simulink model "Group15_Final_Demo_Code"  (R2023a)
settings: Solver=FixedStepAuto  StartTime=0.0  StopTime=inf  FixedStep=0.00001  RelTol=1e-3
undefined symbols (not defined in the file): DiscIntNeverNeededParam
libraries: arduinolib x14, simulink x3, hdlsllib x2, mobileRoboticsTrainingLib x1, arduinosensorlib x1
settings Model: NumberOfSteps=50  PacingRate=1000  ExtModeTrigDuration=2  Creator=Boitumelo  LastModifiedBy=jana
settings OptimizationCC: EnhancedBackFolding=on  PassReuseOutputArgsAs=Individual arguments  ZeroExternalMemoryAtStartup=off  ZeroInternalMemoryAtStartup=off  MaxStackSize=64  OptimizeBlockOrder=speed  DifferentSizesBufferReuse=on  OptimizationCustomize=off  EfficientTunableParamExpr=on
settings DebuggingCC: ParameterTunabilityLossMsg=error  UnconnectedInputMsg=warning  UnconnectedOutputMsg=warning  UnconnectedLineMsg=warning  UnderSpecifiedDimensionMsg=warning
settings HardwareCC: ProdBitPerPointer=32  ProdBitPerSizeT=32  ProdBitPerPtrDiffT=32  ProdLargestAtomicInteger=Long  ProdLargestAtomicFloat=Double  ProdWordSize=32  ProdHWDeviceType=ARM Compatible->ARM Cortex  UseEmbeddedCoderFeatures=off  UseSimulinkCoderFeatures=off
settings ModelReferenceCC: EnableRefExpFcnMdlSchedulingChecks=on
settings SFSimCC: MATLABDynamicMemAlloc=off
settings RTWCC: Description=Embedded Coder  SystemTargetFile=ert.tlc  HardwareBoard=Arduino Nano 33 IoT  TemplateMakefile=ert_default_tmf  Toolchain=Arduino ARM  BuildConfiguration=Faster Runs  DLArmComputeVersion=19.05
settings CodeAppCC: ForceParamTrailComments=on  IgnoreCustomStorageClasses=off  OperatorAnnotations=on  SimulinkDataObjDesc=on  SFDataObjDesc=on  InsertBlockDesc=on
settings ERTTargetCC: SupportContinuousTime=on  SupportNonInlinedSFcns=on  SupportVariableSizeSignals=on  ExtModeTransport=2  ExtModeStaticAlloc=on  ExtModeAutomaticAllocSize=off  ExtModeStaticAllocSize=8192  ExtModeMexFile=ext_xcp  ExtModeIntrfLevel=Level2 - Open

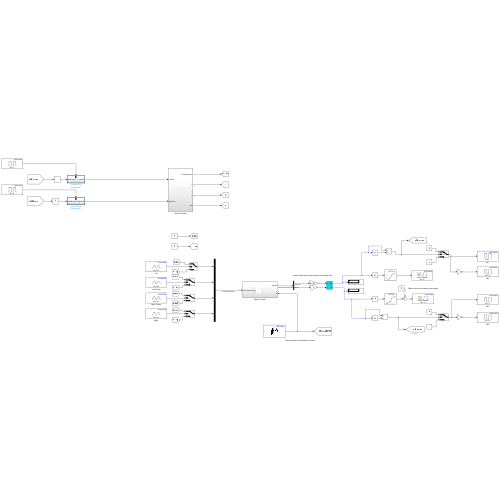
[thumbnail: Simulink's stored preview of the top-level diagram]
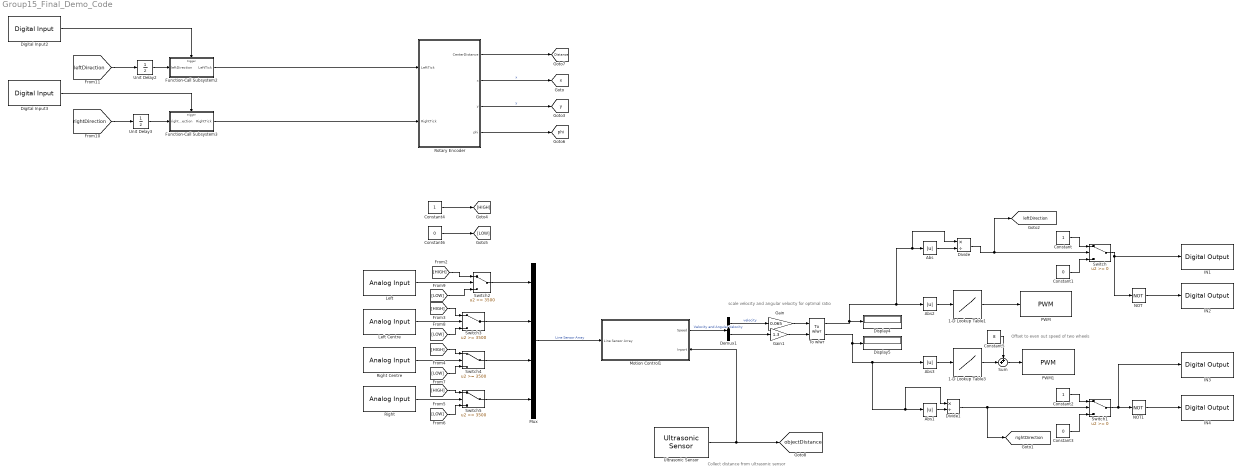
== system Group15_Final_Demo_Code ==
  note: Offset to even out speed of two wheels
  note: Collect distance from ultrasonic sensor
  note: scale velocity and angular velocity for optimal ratio
  1-D Lookup Table1 : Lookup_n-D  NumberOfTableDimensions=1  BreakpointsForDimension1=[-12.5105278523077 -12.3751973907692 -12.2398669292308 -12.1045364676923 -11.9692060061538 -11.8338755446154 -11.6985450830769 -11.5632146215385 -11.42788416 -11.2925536984615 -11.1572232369231 -11.0218927753846 -10.8865623138461 -10.7512318523077 -10.6159013907692 -10.4805709292308 -10.3452404676923 -10.2099100061538 -10.0745795446154 -9.93924908307692 -9.80391862153846 -9.66858816 -9.53325769846154 -9.39792723692308 -9.26259677538462 -9.12726631384615 -8.99193585230769 -8.85660539076923 -8.72127492923077 -8.58594446769231 -8.45061400615385 -8.31528354461539 -8.17995308307692 -8.04462262153846 -7.90929216 -7.77396169846154 -7.63863123692308 -7.50330077538462 -7.36797031384615 -7.23263985230769 -7.09730939076923 -6.96197892923077 -6.82664846769231 -6.69131800615385 -6.55598754461539 -6.42065708307692 -6.28532662153846 -6.14999616 -6.01466569846154 -5.87933523692308 -5.74400477538462 -5.60867431384616 -5.47334385230769 -5.33801339076923 -5.20268292923077 -5.06735246769231 -4.93202200615385 -4.79669154461538 -4.66136108307692 -4.52603062153846 -4.39070016 -4.303992 -4.178328 -4.021248 -3.832752 -3.644256 -3.518592 -3.45576 -3.330096 -3.204432 -3.015936 -2.890272 -2.764608 -2.576112 -2.51328 -2.3562 -2.167704 -2.136288 -1.916376 -1.790712 -1.633632 -1.5708 -1.445136 -1.350888 -1.162392 -1.005312 0 1.005312 1.162392 1.350888 1.445136 1.5708 1.633632 1.790712 1.916376 2.136288 2.167704 2.3562 2.51328 2.576112 2.764608 2.890272 3.015936 3.204432 3.330096 3.45576 3.518592 3.644256 3.832752 4.021248 4.178328 4.303992 4.39070016 4.52603062153846 4.66136108307692 4.79669154461538 4.93202200615384 5.06735246769231 5.20268292923077 5.33801339076923 5.47334385230769 5.60867431384615 5.74400477538461 5.87933523692307 6.01466569846154 6.14999616 6.28532662153846 6.42065708307692 6.55598754461538 6.69131800615384 6.8266484676923 6.96197892923077 7.09730939076923 7.23263985230769 7.36797031384615 7.50330077538461 7.63863123692307 7.77396169846154 7.90929216 8.04462262153846 8.17995308307692 8.31528354461538 8.45061400615384 8.5859444676923 8.72127492923077 8.85660539076923 8.99193585230769 9.12726631384615 9.26259677538461 9.39792723692307 9.53325769846153 9.66858816 9.80391862153846 9.93924908307692 10.0745795446154 10.2099100061538 10.3452404676923 10.4805709292308 10.6159013907692 10.7512318523077 10.8865623138462 11.0218927753847 11.1572232369231 11.2925536984616 11.42788416 11.5632146215385 11.698545083077 11.8338755446154 11.9692060061539 12.1045364676923 12.2398669292308 12.3751973907693 12.5105278523077]  Table=[-127 -126 -125 -124 -123 -122 -121 -120 -119 -118 -117 -116 -115 -114 -113 -112 -111 -110 -109 -108 -107 -106 -105 -104 -103 -102 -101 -100 -99 -98 -97 -96 -95 -94 -93 -92 -91 -90 -89 -88 -87 -86 -85 -84 -83 -82 -81 -80 -79 -78 -77 -76 -75 -74 -73 -72 -71 -70 -69 -68 -67 -66 -65 -64 -63 -62 -61 -60 -59 -58 -57 -56 -55 -54 -53 -52 -51 -50 -49 -48 -47 -46 -45 -44 -43 -42 0 42 43 44 45 46 47 48 49 50 51 52 53 54 55 56 57 58 59 60 61 62 63 64 65 66 67 68 69 70 71 72 73 74 75 76 77 78 79 80 81 82 83 84 85 86 87 88 89 90 91 92 93 94 95 96 97 98 99 100 101 102 103 104 105 106 107 108 109 110 111 112 113 114 115 116 117 118 119 120 121 122 123 124 125 126 127]  InternalRulePriority=Speed  RndMeth=Simplest
  1-D Lookup Table3 : Lookup_n-D  NumberOfTableDimensions=1  BreakpointsForDimension1=[-12.5105278523077 -12.3751973907692 -12.2398669292308 -12.1045364676923 -11.9692060061538 -11.8338755446154 -11.6985450830769 -11.5632146215385 -11.42788416 -11.2925536984615 -11.1572232369231 -11.0218927753846 -10.8865623138461 -10.7512318523077 -10.6159013907692 -10.4805709292308 -10.3452404676923 -10.2099100061538 -10.0745795446154 -9.93924908307692 -9.80391862153846 -9.66858816 -9.53325769846154 -9.39792723692308 -9.26259677538462 -9.12726631384615 -8.99193585230769 -8.85660539076923 -8.72127492923077 -8.58594446769231 -8.45061400615385 -8.31528354461539 -8.17995308307692 -8.04462262153846 -7.90929216 -7.77396169846154 -7.63863123692308 -7.50330077538462 -7.36797031384615 -7.23263985230769 -7.09730939076923 -6.96197892923077 -6.82664846769231 -6.69131800615385 -6.55598754461539 -6.42065708307692 -6.28532662153846 -6.14999616 -6.01466569846154 -5.87933523692308 -5.74400477538462 -5.60867431384616 -5.47334385230769 -5.33801339076923 -5.20268292923077 -5.06735246769231 -4.93202200615385 -4.79669154461538 -4.66136108307692 -4.52603062153846 -4.39070016 -4.303992 -4.178328 -4.021248 -3.832752 -3.644256 -3.518592 -3.45576 -3.330096 -3.204432 -3.015936 -2.890272 -2.764608 -2.576112 -2.51328 -2.3562 -2.167704 -2.136288 -1.916376 -1.790712 -1.633632 -1.5708 -1.445136 -1.350888 -1.162392 -1.005312 0 1.005312 1.162392 1.350888 1.445136 1.5708 1.633632 1.790712 1.916376 2.136288 2.167704 2.3562 2.51328 2.576112 2.764608 2.890272 3.015936 3.204432 3.330096 3.45576 3.518592 3.644256 3.832752 4.021248 4.178328 4.303992 4.39070016 4.52603062153846 4.66136108307692 4.79669154461538 4.93202200615384 5.06735246769231 5.20268292923077 5.33801339076923 5.47334385230769 5.60867431384615 5.74400477538461 5.87933523692307 6.01466569846154 6.14999616 6.28532662153846 6.42065708307692 6.55598754461538 6.69131800615384 6.8266484676923 6.96197892923077 7.09730939076923 7.23263985230769 7.36797031384615 7.50330077538461 7.63863123692307 7.77396169846154 7.90929216 8.04462262153846 8.17995308307692 8.31528354461538 8.45061400615384 8.5859444676923 8.72127492923077 8.85660539076923 8.99193585230769 9.12726631384615 9.26259677538461 9.39792723692307 9.53325769846153 9.66858816 9.80391862153846 9.93924908307692 10.0745795446154 10.2099100061538 10.3452404676923 10.4805709292308 10.6159013907692 10.7512318523077 10.8865623138462 11.0218927753847 11.1572232369231 11.2925536984616 11.42788416 11.5632146215385 11.698545083077 11.8338755446154 11.9692060061539 12.1045364676923 12.2398669292308 12.3751973907693 12.5105278523077]  Table=[-127 -126 -125 -124 -123 -122 -121 -120 -119 -118 -117 -116 -115 -114 -113 -112 -111 -110 -109 -108 -107 -106 -105 -104 -103 -102 -101 -100 -99 -98 -97 -96 -95 -94 -93 -92 -91 -90 -89 -88 -87 -86 -85 -84 -83 -82 -81 -80 -79 -78 -77 -76 -75 -74 -73 -72 -71 -70 -69 -68 -67 -66 -65 -64 -63 -62 -61 -60 -59 -58 -57 -56 -55 -54 -53 -52 -51 -50 -49 -48 -47 -46 -45 -44 -43 -42 0 42 43 44 45 46 47 48 49 50 51 52 53 54 55 56 57 58 59 60 61 62 63 64 65 66 67 68 69 70 71 72 73 74 75 76 77 78 79 80 81 82 83 84 85 86 87 88 89 90 91 92 93 94 95 96 97 98 99 100 101 102 103 104 105 106 107 108 109 110 111 112 113 114 115 116 117 118 119 120 121 122 123 124 125 126 127]  InternalRulePriority=Speed  RndMeth=Simplest
  Abs{,1..3} (4 alike) : Abs  SaturateOnIntegerOverflow=off
  Constant : Constant
  Constant1 : Constant  Value=0
  Constant2 : Constant
  Constant3 : Constant  Value=0
  Constant4 : Constant
  Constant5 : Constant  Value=8
  Constant6 : Constant  Value=0
  Demux1 : Demux  Outputs=2
  Digital Input2 : arduinolib/Digital Input  pinNumber=3  mode=Default  Direction=input  SampleTime=0.001  blockPlatform=arduino
  Digital Input3 : arduinolib/Digital Input  pinNumber=2  mode=Default  Direction=input  SampleTime=0.001  blockPlatform=arduino
  Display4 : Display
  Display5 : Display
  Divide : Product  Inputs=*/
  Divide1 : Product  Inputs=*/
  Function-Call Subsystem2 : Subsystem  TreatAsAtomicUnit=on
  Function-Call Subsystem3 : Subsystem  TreatAsAtomicUnit=on
  Gain : Gain  Gain=0.065
  Gain1 : Gain  Gain=1.3
  IN1 : arduinolib/Digital Output  pinNumber=7  Direction=output  blockPlatform=arduino
  IN2 : arduinolib/Digital Output  pinNumber=8  Direction=output  blockPlatform=arduino
  IN3 : arduinolib/Digital Output  pinNumber=9  Direction=output  blockPlatform=arduino
  IN4 : arduinolib/Digital Output  pinNumber=10  Direction=output  blockPlatform=arduino
  Left : arduinolib/Analog Input  pinNumber=7  ReadResultsOnly=off  ConversionTriggerSource=Software  ExternalTriggerType=uint32( 0 )  OutputDataType=uint16  EnableConversionCompleteNotify=off  EnableOuputStatus=off  SampleTime=0.0001  blockPlatform=arduino
  Left Centre : arduinolib/Analog Input  pinNumber=0  ReadResultsOnly=off  ConversionTriggerSource=Software  ExternalTriggerType=uint32( 0 )  OutputDataType=uint16  EnableConversionCompleteNotify=off  EnableOuputStatus=off  SampleTime=0.0001  blockPlatform=arduino
  Motion Control1 : Subsystem
      settings: PortSchema="{\"entries\":[{\"content\":{\"sides\":[{\"content\":{\"connectorIds\":[\"In1\"]},\"type\":\"ConnectorPlacement.EquallySpacedRectSide\",\"uuid\":\"8c902054-c90d-4041-a30b-e9972f3a80fd\"},{\"content\":{\"connectorIds\":[\"Out1\",\"In2\"],\"side\":\"RIGHT\"},\"type\":\"ConnectorPlacement.EquallySpacedRectSide\",\"uuid\":\"d90cf934-ce11-4f50-afe0-98fc417ab745\"},{\"content\":{\"side\":\"TOP\"},\"type\":\"ConnectorPlacement.EquallySpacedRectSide\",\"uuid\":\"2acc5f33-e61f-44f0-84c4-b841351b747b\"}]},\"type\":\"ConnectorPlacement.EquallySpacedConnector\",\"uuid\":\"ebe61945-3866-4bce-ba54-5c93c237d4bb\"}],\"packageUris\":[\"http://schema.mathworks.com/mf0/Connector/R2020b\"],\"version\":\"1.0\"}"
  Mux : Mux
  NOT : Logic  Operator=NOT  IconShape=distinctive  AllPortsSameDT=off  OutDataTypeStr=boolean
  NOT1 : Logic  Operator=NOT  IconShape=distinctive  AllPortsSameDT=off  OutDataTypeStr=boolean
  PWM : arduinolib/PWM  pinNumber=6  frequencyType=Default  desiredFrequency=490.2  achievableFrequency=490.2
  PWM1 : arduinolib/PWM  pinNumber=11  frequencyType=Default  desiredFrequency=490.2  achievableFrequency=490.2
  Right : arduinolib/Analog Input  pinNumber=2  ReadResultsOnly=off  ConversionTriggerSource=Software  ExternalTriggerType=uint32( 0 )  OutputDataType=uint16  EnableConversionCompleteNotify=off  EnableOuputStatus=off  SampleTime=0.0001  blockPlatform=arduino
  Right Centre : arduinolib/Analog Input  pinNumber=1  ReadResultsOnly=off  ConversionTriggerSource=Software  ExternalTriggerType=uint32( 0 )  OutputDataType=uint16  EnableConversionCompleteNotify=off  EnableOuputStatus=off  SampleTime=0.0001  blockPlatform=arduino
  Rotary Encoder : Subsystem
  Sum : Sum  Inputs=++|
  Switch : Switch  SaturateOnIntegerOverflow=off  InputSameDT=off
  Switch1 : Switch  SaturateOnIntegerOverflow=off  InputSameDT=off
  Switch{2..5} (4 alike) : Switch  Threshold=3500  SaturateOnIntegerOverflow=off  InputSameDT=off
  To wlwr : mobileRoboticsTrainingLib/To wlwr  axleLength=0.17  wheelR=0.031
  Ultrasonic Sensor : arduinosensorlib/Ultrasonic Sensor  NumSignalPins=2  TrigPin=4  EchoPin=5  SignalPin=3  SampleTime_=0.05  blockPlatform=ARDUINO
  Unit Delay2 : UnitDelay  SampleTime=-1  HasFrameUpgradeWarning=on
  Unit Delay3 : UnitDelay  SampleTime=-1  HasFrameUpgradeWarning=on
  tag scope: Distance=global, leftDirection=global, objectDistance=global, phi=global, rightDirection=global, x=global, y=global
  wires:
  Mux/1 -> Motion Control1/1(Line Sensor Array)  "Line Sensor Array"
  Abs/1 -> Divide/2
  Divide/1 -> [leftDirection], Switch/2
  Divide1/1 -> [rightDirection], Switch1/2
  Abs1/1 -> Divide1/2
  Constant/1 -> Switch/1
  Switch/1 -> NOT/1, IN1/1
  Constant1/1 -> Switch/3
  NOT/1 -> IN2/1
  Constant2/1 -> Switch1/1
  Switch1/1 -> NOT1/1, IN3/1
  Constant3/1 -> Switch1/3
  NOT1/1 -> IN4/1
  [HIGH] -> Switch2/1
  [HIGH] -> Switch3/1
  [HIGH] -> Switch4/1
  [HIGH] -> Switch5/1
  [LOW] -> Switch5/3
  [LOW] -> Switch4/3
  [LOW] -> Switch3/3
  [LOW] -> Switch2/3
  Left/1 -> Switch2/2
  Right Centre/1 -> Switch4/2
  Right/1 -> Switch5/2
  Switch2/1 -> Mux/1
  Switch3/1 -> Mux/2
  Switch4/1 -> Mux/3
  Switch5/1 -> Mux/4
  Constant4/1 -> [HIGH]
  Constant6/1 -> [LOW]
  1-D Lookup Table1/1 -> PWM/1
  1-D Lookup Table3/1 -> Sum/2
  Ultrasonic Sensor/1 -> Motion Control1/2(Inport), [objectDistance]
  [rightDirection] -> Unit Delay3/1
  Unit Delay3/1 -> Function-Call Subsystem3/1(rightDirection)
  Unit Delay2/1 -> Function-Call Subsystem2/1(leftDirection)
  Rotary Encoder/3(y) -> [y]  "y"
  Rotary Encoder/2(x) -> [x]  "x"
  Digital Input3/1 -> Function-Call Subsystem3/Trigger
  Digital Input2/1 -> Function-Call Subsystem2/Trigger
  [leftDirection] -> Unit Delay2/1
  Function-Call Subsystem2/1(LeftTick) -> Rotary Encoder/1(LeftTick)
  Rotary Encoder/4(phi) -> [phi]
  Function-Call Subsystem3/1(RightTick) -> Rotary Encoder/2(RightTick)
  Left Centre/1 -> Switch3/2
  Rotary Encoder/1(CenterDistance) -> [Distance]
  To wlwr/1 -> Divide/1, Abs/1, Abs2/1, Display4/1
  To wlwr/2 -> Abs3/1, Divide1/1, Abs1/1, Display5/1
  Abs2/1 -> 1-D Lookup Table1/1
  Abs3/1 -> 1-D Lookup Table3/1
  Constant5/1 -> Sum/1
  Sum/1 -> PWM1/1
  Gain/1 -> To wlwr/1
  Gain1/1 -> To wlwr/2
  Motion Control1/1(Speed) -> Demux1/1  "Velocity and Angular Velocity"
  Demux1/2 -> Gain1/1
  Demux1/1 -> Gain/1  "velocity"

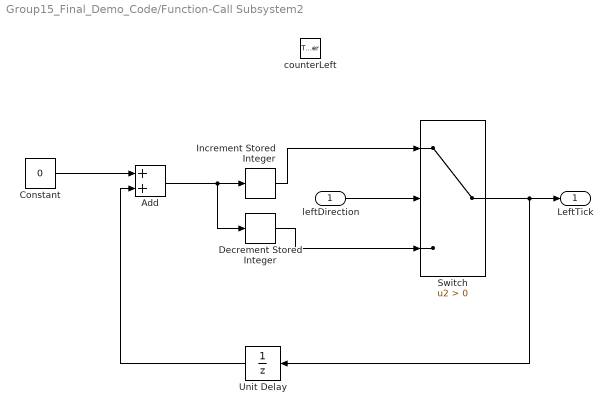
== system Group15_Final_Demo_Code/Function-Call Subsystem2 ==
  leftDirection : Inport
  counterLeft : TriggerPort  TriggerType=falling  FunctionName=counterLeft  VariantControl=(inherit)
  Add : Sum
  Constant : Constant  Value=0
  Decrement Stored Integer : simulink/Additional Math & Discrete/Additional Math: Increment - Decrement/Decrement Stored Integer
  Increment Stored Integer : hdlsllib/Math Operations/Increment Stored Integer
  Switch : Switch  Criteria=u2 > Threshold  SaturateOnIntegerOverflow=off  InputSameDT=off
  Unit Delay : UnitDelay  SampleTime=-1  HasFrameUpgradeWarning=on
  LeftTick : Outport
  wires:
  Decrement Stored Integer/1 -> Switch/3
  Increment Stored Integer/1 -> Switch/1
  Unit Delay/1 -> Add/2
  leftDirection/1 -> Switch/2
  Constant/1 -> Add/1
  Switch/1 -> Unit Delay/1, LeftTick/1
  Add/1 -> Decrement Stored Integer/1, Increment Stored Integer/1

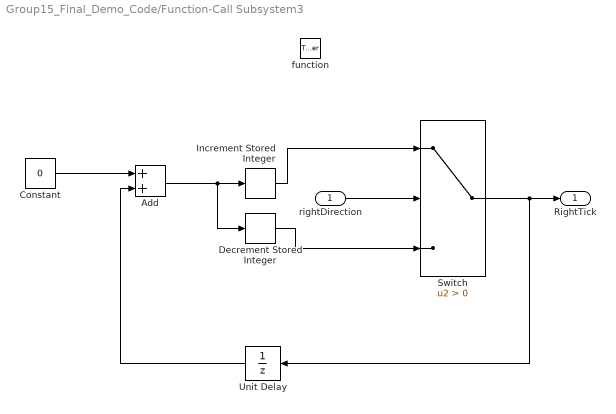
== system Group15_Final_Demo_Code/Function-Call Subsystem3 ==
  rightDirection : Inport
  function : TriggerPort  TriggerType=falling  VariantControl=(inherit)
  Add : Sum
  Constant : Constant  Value=0
  Decrement Stored Integer : simulink/Additional Math & Discrete/Additional Math: Increment - Decrement/Decrement Stored Integer
  Increment Stored Integer : hdlsllib/Math Operations/Increment Stored Integer
  Switch : Switch  Criteria=u2 > Threshold  SaturateOnIntegerOverflow=off  InputSameDT=off
  Unit Delay : UnitDelay  SampleTime=-1  HasFrameUpgradeWarning=on
  RightTick : Outport
  wires:
  Decrement Stored Integer/1 -> Switch/3
  Increment Stored Integer/1 -> Switch/1
  Unit Delay/1 -> Add/2
  rightDirection/1 -> Switch/2
  Constant/1 -> Add/1
  Switch/1 -> Unit Delay/1, RightTick/1
  Add/1 -> Decrement Stored Integer/1, Increment Stored Integer/1

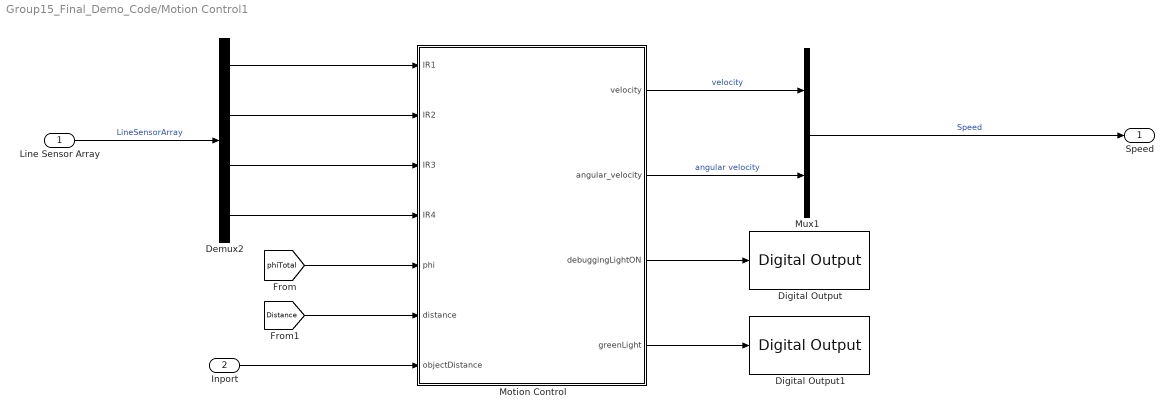
== system Group15_Final_Demo_Code/Motion Control1 ==
  Line Sensor Array : Inport
  Inport : Inport  Port=2
  Demux2 : Demux
  Digital Output : arduinolib/Digital Output  pinNumber=12  Direction=output  blockPlatform=arduino
  Digital Output1 : arduinolib/Digital Output  pinNumber=0  Direction=output  blockPlatform=arduino
  Motion Control : Stateflow chart  TreatAsAtomicUnit=on  SystemSampleTime=0.001
  Mux1 : Mux  Inputs=2
  Speed : Outport
  wires:
  Line Sensor Array/1 -> Demux2/1  "LineSensorArray"
  Mux1/1 -> Speed/1  "Speed"
  Demux2/1 -> Motion Control/1(IR1)
  Demux2/2 -> Motion Control/2(IR2)
  Demux2/3 -> Motion Control/3(IR3)
  Demux2/4 -> Motion Control/4(IR4)
  [phiTotal] -> Motion Control/5(phi)
  [Distance] -> Motion Control/6(distance)
  Inport/1 -> Motion Control/7(objectDistance)
  Motion Control/1(velocity) -> Mux1/1  "velocity"
  Motion Control/2(angular_velocity) -> Mux1/2  "angular velocity"
  Motion Control/3(debuggingLightON) -> Digital Output/1
  Motion Control/4(greenLight) -> Digital Output1/1

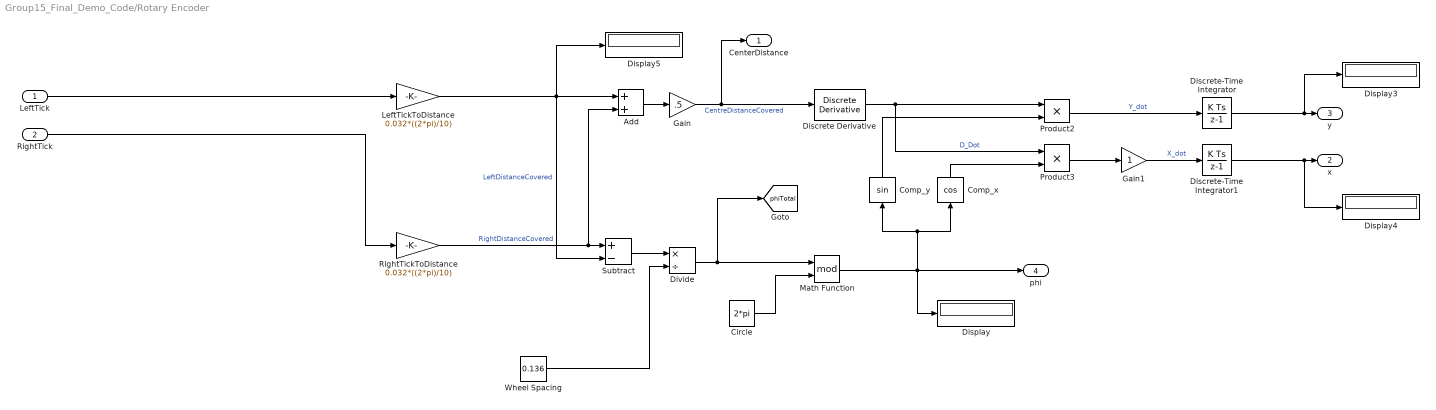
== system Group15_Final_Demo_Code/Rotary Encoder ==
  LeftTick : Inport
  RightTick : Inport  Port=2
  Add : Sum
  Circle : Constant  Value=2*pi
  Comp_x : Trigonometry  Operator=cos
  Comp_y : Trigonometry
  Discrete Derivative : simulink/Discrete/Discrete Derivative  gainval=1.0  ICPrevScaledInput=0.0  OutMin=[]  OutMax=[]  OutDataType=fixdt(1, 16)  OutScaling=2^-10  DoSatur=off
  Discrete-Time Integrator : DiscreteIntegrator  SampleTime=-1  ICPrevOutput=DiscIntNeverNeededParam  ICPrevScaledInput=DiscIntNeverNeededParam
  Discrete-Time Integrator1 : DiscreteIntegrator  SampleTime=-1  ICPrevOutput=DiscIntNeverNeededParam  ICPrevScaledInput=DiscIntNeverNeededParam
  Display{,3..5} (4 alike) : Display
  Divide : Product  Inputs=*/
  Gain : Gain  Gain=.5
  Gain1 : Gain
  LeftTickToDistance : Gain  Gain=0.032*((2*pi)/10)
  Math Function : Math  Operator=mod  SignedPower=on
  Product2 : Product
  Product3 : Product
  RightTickToDistance : Gain  Gain=0.032*((2*pi)/10)
  Subtract : Sum  Inputs=+-
  Wheel Spacing : Constant  Value=0.136
  CenterDistance : Outport
  x : Outport  Port=2
  y : Outport  Port=3
  phi : Outport  Port=4
  tag scope: phiTotal=global
  wires:
  Divide/1 -> [phiTotal], Math Function/1
  Gain/1 -> Discrete Derivative/1, CenterDistance/1  "CentreDistanceCovered"
  Subtract/1 -> Divide/1
  Add/1 -> Gain/1
  RightTickToDistance/1 -> Add/2, Subtract/1  "RightDistanceCovered"
  RightTick/1 -> RightTickToDistance/1
  LeftTickToDistance/1 -> Subtract/2, Add/1, Display5/1  "LeftDistanceCovered"
  Comp_y/1 -> Product2/2
  Comp_x/1 -> Product3/2
  LeftTick/1 -> LeftTickToDistance/1
  Product2/1 -> Discrete-Time Integrator/1  "Y_dot"
  Product3/1 -> Gain1/1
  Wheel Spacing/1 -> Divide/2
  Circle/1 -> Math Function/2
  Discrete Derivative/1 -> Product2/1, Product3/1  "D_Dot"
  Gain1/1 -> Discrete-Time Integrator1/1  "X_dot"
  Math Function/1 -> phi/1, Comp_x/1, Comp_y/1, Display/1
  Discrete-Time Integrator1/1 -> Display4/1, x/1
  Discrete-Time Integrator/1 -> Display3/1, y/1

== stateflow chart Group15_Final_Demo_Code/Motion Control1/Motion Control ==
  note: Basic Description
      | Default: Curve Navigation controls the velocity and angular velocity
      |
      | When infrared sensor 1 or 4 (IR1 and IR4) detect a black line, this Intersection Navigation subsystem takes control and calls the leftTurn or rightTurn procedure respectively.
      | Intersection procedure (same for both leftTurn or rightTurn):
      | 	Increment branchCounter to keep track of the number of branches.
      | 	Move forward a small distance to align with the turn.
      | 	Rotate in the correct direction until the middle two sensors detect a line again.
      | 	Pass control to Curve Navigation to navigate the offshoot.
      | 	If the offshoot comes to an end (all sensors detect white), rotate 180 degrees and navigate back to the main path.
      | 	If the offshoot ends in a detect line (all sensors detect black), stop, send a signal to the Object Detection subsystem to measure for an object, rotate 180 degrees and navigate back to the main path.
      | 		Add branch number from branchCounter to objectMap to indicate this branch has an object.
      | 	Pass control to Curve Navigation to navigate the offshoot returning to the main path.
      | 	When the peripheral sensors detect a black line again (meaning the robot has returned to the intersection with the main branch), control is passed to Intersection Navigation.
      | 	Move forward a small distance to align with the turn.
      | 	Rotate in the correct direction until the middle two sensors detect a line again.
      | 	Pass control back to Curve Navigation to continue traversing the main path.
      |
      | If all sensors detect black whilst the robot is on the main path, the endOfMaze procedure is called.
      | endOfMaze procedure:
      | 	Stop
      | 	Use objectMap to determine how many objects were discovered.
      | 	Find the branch number of the object with the smallest distance, saved to branchWithObject.
      | 		objectCounter provides number of object with smallest distance measured.
      | 		Obtain the n'th number in objectMap to determine the branch number containing said object (where n = objectCounter)
      | 	Invert branchWithObject such that it provides the number of the branch starting from the end of the maze.
      | 	Set renavigating to HIGH.
      |
      | Renavigating Procedure:
      | 	Rotate 180 degrees to re-traverse the maze.
      | 	set branchCounter to 0.
      | 	Pass control to Curve Navigation to renavigate maze.
      | 	If intersection is detected, increment branchCounter.
      | 	If branchCounter is equal to branchWithObject at an intersection, turn into that offshoot.
      | 	Pass control to Curve Navigation to navigate offshoot.
      | 	If all sensors detect black at the "detect object line", come to a stop.
  state deadEnd
    entry: branchNumber = branchNumber + branchfactor;
    state moveForward
      entry: distance0 = distance;
      velocity = 2;
    state Rotate
      velocity = 0;
      angular_velocity = 1.5;
    (default) -> deadEnd.moveForward
    deadEnd.moveForward -> deadEnd.Rotate : [abs(distance - distance0) >= 0.09]
  state moveForward1
    %move forward past intersection
    velocity = 2;
    angular_velocity = 0;
  state moveForward
    %move forward past intersection
    entry: velocity = 2;
    angular_velocity = 0;
  state lineFollowing
    %block that controls line following
    entry:
    distance0 = distance;
    exit: angular_velocity = 0;
    state FollowTrack
      %middle two sense black
      velocity = 2;
      angular_velocity = 0;
    state TurnRight
      entry:
      phi0 = phi;
      velocity = 2;
      angular_velocity = 1.2;
    state TurnLeft
      entry:
      phi0 = phi;
      velocity = 2;
      angular_velocity = -1.2;
    (default) -> FollowTrack
    FollowTrack -> TurnLeft [order 1] : %right middle sensor detects white
        | [IR3 == 1]
    TurnRight -> FollowTrack : %both centred sensors detect black
        | [IR3 == 0 && IR2 == 0]
    FollowTrack -> TurnRight [order 2] : %left middle sensor detects white
        | [IR2 == 1]
    TurnLeft -> FollowTrack : %middle two sensors detect black
        | [IR3 == 0 && IR2 == 0]
  state turnLeft
    entry: lastTurn = 1;
    phi0 = phi;
    during:
    %safety mechanism to combat accidental 'turning on main' turns instead of 'turning onto a branch'
    if IR4 == 0 && mainPathTurn == 1
    onBranch = 1;
    mainPathTurn = 0;
    end
    state moveForward
      entry: velocity = 2;
    state firstRotate
      entry:
      velocity = 0;
      angular_velocity = -1.5;
    state rotateOntoPath
    state rotateOffPath
      %entry:
      %velocity = 0;
      %angular_velocity = -10;
    (default) -> turnLeft.moveForward
    turnLeft.moveForward -> turnLeft.firstRotate : [IR1 == 1]
    turnLeft.firstRotate -> turnLeft.rotateOffPath : [IR1 == 0]
    turnLeft.rotateOffPath -> turnLeft.rotateOntoPath : [IR2 == 1 && IR3 == 1]
  state turnRight
    entry: lastTurn = 2;
    phi0 = phi;
    during:
    %safety mechanism to combat accidental 'turning on main' turns instead of 'turning onto a branch'
    if IR1 == 0 && mainPathTurn == 1
    onBranch = 1;
    mainPathTurn = 0;
    end
    state moveForward
      velocity = 2;
    state firstRotate
      entry:
      velocity = 0;
      angular_velocity = 1.5;
    state rotateOntoPath
    state rotateOffPath
    (default) -> turnRight.moveForward
    turnRight.moveForward -> turnRight.firstRotate : [IR4 == 1]
    turnRight.firstRotate -> turnRight.rotateOffPath : [IR4 == 0]
    turnRight.rotateOffPath -> turnRight.rotateOntoPath : [IR2 == 1 && IR3 == 1]
  state determineIntersection
    %enter when either peripheral sensor detects black
    %move forward to confirm intersection type
    state moveForward
      entry: distance0 = distance;
    state chooseIntersection
      entry: velocity = 0;
    (default) -> determineIntersection.moveForward
    determineIntersection.moveForward -> (junction 1093) : [abs(distance - distance0) >= 0.05]
    (junction 1093) -> chooseIntersection
  state renavIgnore1
    %if busy renavigating, determine
    %if branch should be
    %ignored
  state renavIgnore
    %if busy renavigating, determine
    %if branch should be
    %ignored
  state endOfMaze
    %move forward slightly
    %start counting down branches
    %back to branch with closest object
    entry: distance0 = distance
    branchfactor = -1;
    angular_velocity = 0;
  state Rotate
    %rotate 180 degrees
    entry: phi0 = phi;
    during:
    velocity = 0;
    angular_velocity = 1.2;
  state detectObject
    entry: debuggingLightON = 1;
    exit: debuggingLightON = 0;
    state DoNothing
    state UpdateClosestObj
      entry:
      closestObj = objectDistance;
      returnBranch = branchNumber;
    (default) -> DoNothing
    DoNothing -> UpdateClosestObj [order 1] : %if first object or closer than previous closest object, update closest object
        | [(objectDistance < closestObj && objectDistance ~=0) || branchNumber == 1]
  state FoundHome
    %enter upon renavigating
    %to closest object
  state turnAround
    entry:
    turnAround = 1;
    state moveForward
      entry: distance0 = distance;
      velocity = 2;
    state Rotate
      %rotate 180 degrees
      entry: phi0 = phi;
      during:
      velocity = 0;
      angular_velocity = -1.5;
    (default) -> turnAround.moveForward
    turnAround.moveForward -> turnAround.Rotate : [abs(distance - distance0) >= 0.015]
  deadEnd.Rotate -> lineFollowing : %robot realigns with line
      | [IR2 == 0 && IR3 == 0]{turnAround = 1;}
  lineFollowing -> deadEnd [order 3] : %all sensors detect white
      | [IR1 + IR2 + IR3 + IR4 == 4]
  (default) -> lineFollowing
  (junction 1127) -> moveForward
  (junction 1126) -> (junction 1127) : %decrement branch counter
      | {onBranch = 0, branchNumber = branchNumber + branchfactor;}
  moveForward -> lineFollowing : [IR4 == 1]
  (junction 1112) -> moveForward1
  moveForward1 -> lineFollowing : [IR1 == 1]
  (junction 1110) -> (junction 1112) : %decrement branch counter
      | {onBranch = 0, branchNumber = branchNumber + branchfactor;}
  turnRight.rotateOntoPath -> lineFollowing : %orientated back onto a path
      | [(IR2 == 0 || IR3 == 0) && abs(phi0 - phi) >= 1.3 && IR4 == 1]{turnAround = 0;}
  turnLeft.rotateOntoPath -> lineFollowing : %orientated onto a path
      | [(IR2 == 0 || IR3 == 0) && abs(phi0 - phi) >= 1.3 && IR1 == 1]{turnAround = 0;}
  (junction 1090) -> lineFollowing
  Rotate -> (junction 1090) : %stop turning once realigned with path
      | [abs(phi - phi0) >= 2.6 && IR3 == 0]
  lineFollowing -> determineIntersection [order 2] : [abs(distance0 - distance) >= 0.02 && IR1 == 0]{leftBranch = 1;}
  lineFollowing -> determineIntersection [order 1] : [abs(distance0 - distance) >= 0.02 && IR4 == 0]{rightBranch = 1;}
  (junction 932) -> lineFollowing : %realigned with path
      | [abs(phi - phi0) >= 2.6 &&  IR3 == 0]
  (junction 1103) -> turnLeft
  (junction 1013) -> (junction 1103)
  (junction 1101) -> turnLeft [order 1] : %if branch with final object, turn down branch
      | [branchNumber == returnBranch]{complete =1}
  (junction 900) -> turnLeft : %{branchNumber = branchNumber + branchfactor}
  (junction 950) -> turnLeft
  (junction 948) -> turnRight
  (junction 1123) -> turnRight
  (junction 1015) -> turnRight
  (junction 1119) -> turnRight [order 2] : %if branch with final object, turn down branch
      | [branchNumber == returnBranch]{complete =1}
  chooseIntersection -> (junction 948) [order 5] : %leaving branch, back to main
      | [turnAround == 1 && lastTurn == 2]{onBranch = 0, rightBranch = 0, leftBranch = 0;}
  chooseIntersection -> (junction 950) [order 4] : %leaving branch, return to main
      | [turnAround == 1 && lastTurn == 1]{leftBranch = 0, rightBranch = 0, onBranch = 0;}
  renavIgnore1 -> (junction 1123) [order 1] : %if not renavigating, turn down branch
      | [branchfactor ==1]
  chooseIntersection -> renavIgnore1 [order 2] : %right branch
      | [rightBranch == 1 && leftBranch == 0 && turnAround == 0]{rightBranch = 0, leftBranch = 0, onBranch = 1;}
  renavIgnore -> (junction 900) [order 1] : %if not renavigating, turn down branch
      | [branchfactor ==1]
  chooseIntersection -> renavIgnore [order 3] : %left branch
      | [leftBranch == 1 && rightBranch == 0 && turnAround == 0]{leftBranch = 0, rightBranch = 0, onBranch = 1;}
  renavIgnore1 -> (junction 1141) [order 2] : %if renavigating
      | [branchfactor == -1]
  (junction 1101) -> (junction 1110) [order 2] : %if not branch with final object, ignore and count down
      | [branchNumber ~= returnBranch]
  renavIgnore -> (junction 1101) [order 2] : %if renavigating
      | [branchfactor == -1]
  chooseIntersection -> (junction 1015) [order 1] : %main path turn
      | [IR1 + IR2 + IR3 + IR4 == 4 && rightBranch == 1 && leftBranch == 0 && onBranch == 0]{rightBranch = 0, leftBranch = 0, mainPathTurn = 1;}
  chooseIntersection -> (junction 1139) [order 6]
  determineIntersection -> detectObject [order 2] : %intersection was detected on a branch before turning around, making it a detect line
      | [onBranch == 1 && turnAround == 0]{angular_velocity = 0, velocity = 0, branchNumber = branchNumber + branchfactor;}
  determineIntersection -> endOfMaze [order 1] : %all detect black and on main path
      | [IR1 + IR2 + IR3 + IR4 == 0 && onBranch == 0 && turnAround == 0] {leftBranch = 0, rightBranch = 0;}
  (junction 1141) -> (junction 1119)
  (junction 1119) -> (junction 1126) [order 1] : %if not branch with final object, count down and move past
      | [branchNumber ~= returnBranch]
  (junction 1139) -> (junction 1013) : %main path turn
      | [IR1 + IR2 + IR3 + IR4 == 4 && leftBranch == 1 && rightBranch == 0 && onBranch == 0]{leftBranch = 0, rightBranch = 0, mainPathTurn = 1;}
  endOfMaze -> Rotate : [abs(distance0 - distance) >= 0.03]
  detectObject -> FoundHome : [complete ==1]
  DoNothing -> turnAround [order 2] : %do not update if object not closest
      | after(10, msec)[complete == 0]
  UpdateClosestObj -> turnAround : %update if closest object measured so far
      | [complete == 0 && after(10,msec)||objectDistance ~=0]{turnAround = 1;}
  turnAround.Rotate -> (junction 932)
  data: velocity output; angular_velocity output; IR1 input; IR2 input; IR3 input; IR4 input; phi input; phi0 local; distance input; distance0 local =0; turnAround local =0; objectDistance input; lastTurn local =0; leftBranch local =0; rightBranch local =0; closestObj local =2; branchNumber local =0; branchfactor local =1; returnBranch local =0; debuggingLightON output =0; onBranch local =0; greenLight output =0; complete local =0; mainPathTurn local =0
